simulink model "System"  (R2018a)
settings: Solver=VariableStepAuto  StartTime=0.0  StopTime=10.0  RelTol=1e-3
InitFcn:
  | %Load track data generated by 'parse_track.py'
  | load("track_data")
  | 
  | %Set initial position and pose of Car
  | c_init_x = 0;
  | c_init_y = 0;
  | c_init_theta = 0;
settings Model: Creator=Alex  LastModifiedBy=Alex

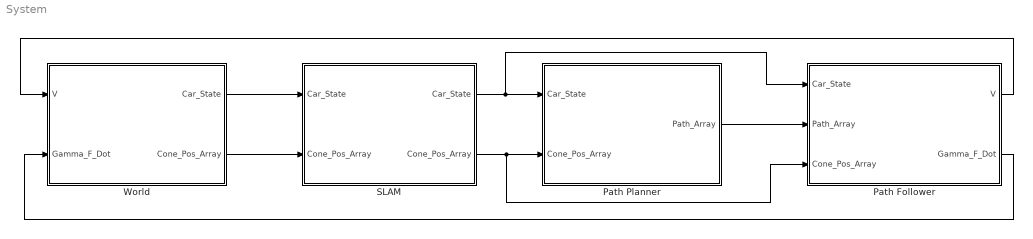
== system System ==
  Path Follower : Subsystem
  Path Planner : Subsystem
  SLAM : Subsystem
  World : Subsystem
  wires:
  Path Follower/1(V) -> World/1(V)
  Path Follower/2("Gamma_F_Dot ") -> World/2("Gamma_F_Dot ")
  Path Planner/1(Path_Array) -> Path Follower/2("Path_Array ")
  SLAM/2(Cone_Pos_Array) -> Path Follower/3(Cone_Pos_Array), Path Planner/2(Cone_Pos_Array)
  SLAM/1("Car_State ") -> Path Follower/1("Car_State "), Path Planner/1(Car_State)
  World/2(Cone_Pos_Array) -> SLAM/2("Cone_Pos_Array ")
  World/1(Car_State) -> SLAM/1(Car_State)

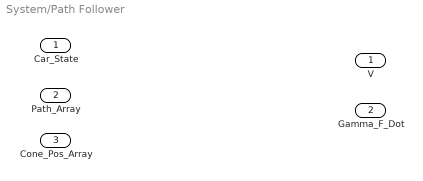
== system System/Path Follower ==
  "Car_State " : Inport
  "Path_Array " : Inport  Port=2
  Cone_Pos_Array : Inport  Port=3
  V : Outport
  "Gamma_F_Dot " : Outport  Port=2

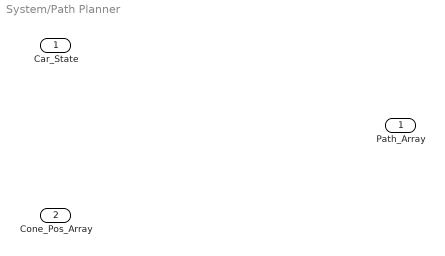
== system System/Path Planner ==
  Car_State : Inport
  Cone_Pos_Array : Inport  Port=2
  Path_Array : Outport

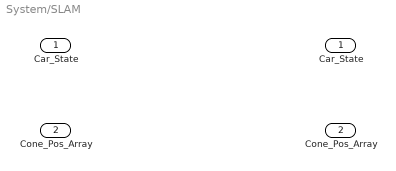
== system System/SLAM ==
  Car_State : Inport
  "Cone_Pos_Array " : Inport  Port=2
  "Car_State " : Outport
  Cone_Pos_Array : Outport  Port=2

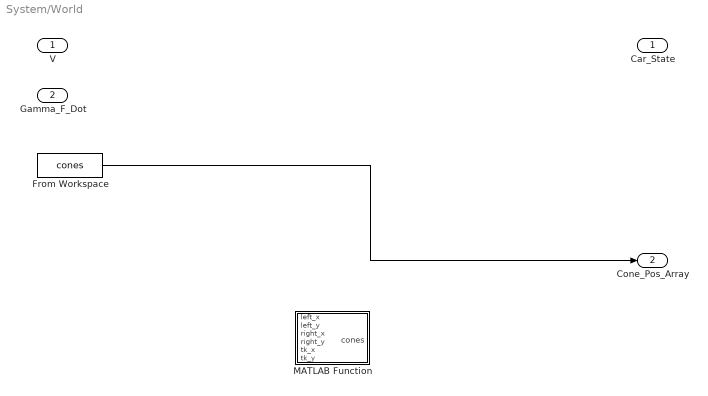
== system System/World ==
  V : Inport
  "Gamma_F_Dot " : Inport  Port=2
  From Workspace : FromWorkspace  VariableName=cones  SampleTime=0
  MATLAB Function : MATLAB Function  TreatAsAtomicUnit=on
  Car_State : Outport
  Cone_Pos_Array : Outport  Port=2
  wires:
  From Workspace/1 -> Cone_Pos_Array/1

== matlab function System/World/MATLAB Function ==
  data: left_x input; cones output; left_y input; right_x input; right_y input; tk_x input; tk_y input
function cones = fcn(left_x,left_y,right_x,right_y,tk_x,tk_y)

    i = 1;
    cones = Cone.empty;
    for j = 1:numel(left_x)
        cones(i) = Cone(left_x(j),left_y(j),'b');
        i=i+1;
    end

    for j = 1:numel(right_x)
        cones(i) = Cone(right_x(j),right_y(j),'y');
        i=i+1;
    end

    for j = 1:numel(tk_x)
        cones(i) = Cone(tk_x(j),tk_y(j),'r');
        i=i+1;
    end
end
